simulink model "PX31s"  (R2015b)
settings: Solver=VariableStepAuto  StartTime=0.0  StopTime=5  RelTol=1e-3
settings Model: Creator=xmax1946  LastModifiedBy=xmax1946

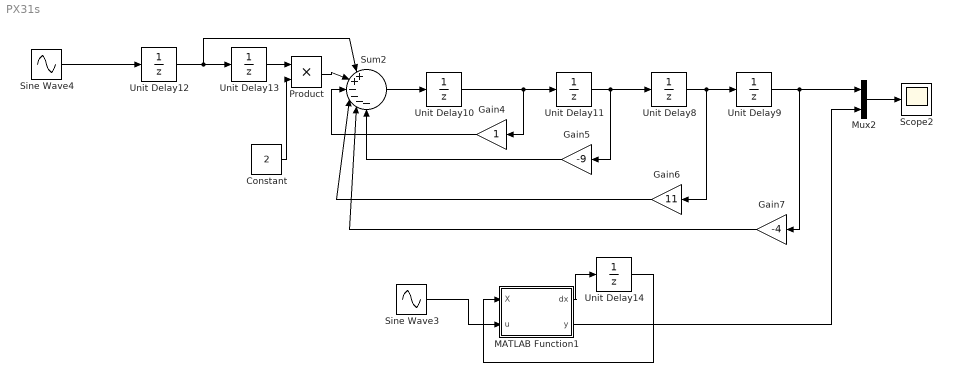
== system PX31s ==
  Constant : Constant  Value=2  SampleTime=1
  Gain4 : Gain
  Gain5 : Gain  Gain=-9
  Gain6 : Gain  Gain=11
  Gain7 : Gain  Gain=-4
  MATLAB Function1 : MATLAB Function  TreatAsAtomicUnit=on
  Mux2 : Mux  Inputs=2
  Product : Product
  Scope2 : Scope
  Sine Wave3 : Sin  Samples=1  SampleTime=1
  Sine Wave4 : Sin  Phase=4  Samples=1  SampleTime=1
  Sum2 : Sum  Inputs=|++----
  Unit Delay10 : UnitDelay  InitialCondition=51.2788  SampleTime=-1
  Unit Delay11 : UnitDelay  InitialCondition=-9.7905  SampleTime=-1
  Unit Delay12 : UnitDelay  InitialCondition=sin(3)  SampleTime=-1
  Unit Delay13 : UnitDelay  InitialCondition=sin(2)  SampleTime=-1
  Unit Delay14 : UnitDelay  InitialCondition=[1;2;-1;-3]  SampleTime=-1
  Unit Delay8 : UnitDelay  InitialCondition=5.408  SampleTime=-1
  Unit Delay9 : UnitDelay  InitialCondition=1.6480  SampleTime=-1
  wires:
  Mux2/1 -> Scope2/1
  Unit Delay10/1 -> Unit Delay11/1, Gain4/1
  Sum2/1 -> Unit Delay10/1
  Gain4/1 -> Sum2/3
  Unit Delay11/1 -> Gain5/1, Unit Delay8/1
  Unit Delay8/1 -> Gain6/1, Unit Delay9/1
  Unit Delay9/1 -> Gain7/1, Mux2/1
  Gain6/1 -> Sum2/4
  Gain7/1 -> Sum2/5
  Gain5/1 -> Sum2/6
  Unit Delay12/1 -> Sum2/1, Unit Delay13/1
  MATLAB Function1/1(dx) -> Unit Delay14/1
  Unit Delay14/1 -> MATLAB Function1/1(X)
  MATLAB Function1/2(y) -> Mux2/2
  Sine Wave4/1 -> Unit Delay12/1
  Sine Wave3/1 -> MATLAB Function1/2(u)
  Unit Delay13/1 -> Product/1
  Product/1 -> Sum2/2
  Constant/1 -> Product/2

== matlab function PX31s/MATLAB Function1 ==
  data: X input; dx output; u input; y output
function [dx,y]= fcn(X,u)


A=[1,1,0,0
    0,1,1,0
    0,0,1,0
    0,0,0,-4];
B=[0;0;1;1];
C=[.6,1.28,.744,.256];

dx=A*X+B*u;
y=C*X;

% [-0.0379;1.9455;-4.5769;6.5769]
% [-8.8993;-6.1657,-1.8636,.4839]
% [-4.231;-2.7423;-.7343;.3056]
% [-37.9663;-24.1346;-9.4423;-1.1538]
%   [-27.3125;-16.3864;-5.5682;-0.2929]
% [-27.5625;-16.5682;-5.6591;-0.3131]
% [-49.1250;-32.25;-13.5;-2.0556]
% [-49.2826;-32.5057;-13.9830;-2.3763]
